simulink model "FSAC2021"  (R2014a)
settings: Solver=FixedStepDiscrete  StartTime=0.0  StopTime=inf  FixedStep=0.0005  RelTol=1e-3
model workspace (MAT data in the model file):
  MCOS : class17 (value not decoded)
  MCOS : class17 (value not decoded)
  MCOS : class17 (value not decoded)
  MCOS : class17 (value not decoded)
  MCOS : class17 (value not decoded)
  MCOS : class17 (value not decoded)
  MCOS : class17 (value not decoded)
  MCOS : class17 (value not decoded)
  MCOS : class17 (value not decoded)
  MCOS : class17 (value not decoded)
  MCOS : class17 (value not decoded)
  MCOS : class17 (value not decoded)
  MCOS : class17 (value not decoded)
  MCOS : class17 (value not decoded)
  MCOS : class17 (value not decoded)
  MCOS : class17 (value not decoded)
  MCOS : class17 (value not decoded)
  MCOS : class17 (value not decoded)
  MCOS : class17 (value not decoded)
  BUZZER_START = 1
  MCOS : class17 (value not decoded)
  MCOS : class17 (value not decoded)
  MCOS : class17 (value not decoded)
  MCOS : class17 (value not decoded)
  MCOS : class17 (value not decoded)
  MCOS : class17 (value not decoded)
  MCOS : class17 (value not decoded)
  MCOS : class17 (value not decoded)
  MCOS : class17 (value not decoded)
  MCOS : class17 (value not decoded)
  MCOS : class17 (value not decoded)
  MCOS : class17 (value not decoded)
  MCOS : class17 (value not decoded)
  MCOS : class17 (value not decoded)
  MCOS : class17 (value not decoded)
  MCOS : class17 (value not decoded)
  MCOS : class17 (value not decoded)
  MCOS : class17 (value not decoded)
  MCOS : class17 (value not decoded)
  MCOS : class17 (value not decoded)
  MCOS : class17 (value not decoded)
  MCOS : class17 (value not decoded)
  MCOS : class17 (value not decoded)
  MCOS : class17 (value not decoded)
  MCOS : class17 (value not decoded)
  MCOS : class17 (value not decoded)
  MCOS : class17 (value not decoded)
  MCOS : class17 (value not decoded)
  MCOS : class17 (value not decoded)
  MCOS : class17 (value not decoded)
  MCOS : class17 (value not decoded)
  MCOS : class17 (value not decoded)
  MCOS : class17 (value not decoded)
  MCOS : class17 (value not decoded)
  MCOS : class17 (value not decoded)
  MCOS : class17 (value not decoded)
  MCOS : class17 (value not decoded)
  MCOS : class17 (value not decoded)
  Brake = 11
  MCOS : class17 (value not decoded)
  MCOS : class17 (value not decoded)
  MCOS : class17 (value not decoded)
  MCOS : class17 (value not decoded)
  MCOS : class17 (value not decoded)
  MCOS : class17 (value not decoded)
  MCOS : class17 (value not decoded)
  MCOS : class17 (value not decoded)
  Sensor_Acc_b = 101.85
  Sensor_Acc_k = -0.0185
  Str_Sen_Orig_Angle = -341
  MCOS : class17 (value not decoded)
  Tire_D = 0.47
  T = 0.05
libraries: simulink x396, ec55xxlib x126
(part 2 of 17)

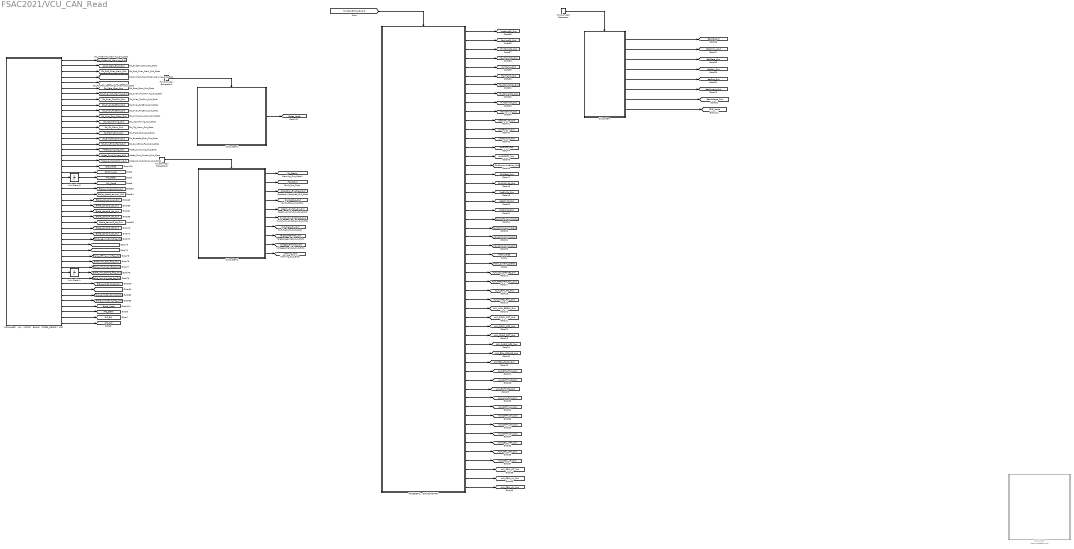
== system FSAC2021/VCU_CAN_Read ==
  DCAN_REC : Subsystem  Commented=on
  Function-Call Generator : simulink/Ports & Subsystems/Function-Call Generator  sample_time=0.1  numberOfIterations=1
  Function-Call Generator1 : simulink/Ports & Subsystems/Function-Call Generator  sample_time=0.5  numberOfIterations=1
  Function-Call Generator2 : simulink/Ports & Subsystems/Function-Call Generator  sample_time=0.1  numberOfIterations=1
  PCANA(RES、AMI、MOTEC、BRAKE、STEER_SENSOR、IPC) : Subsystem
  PCANB(BMS、DRIVE_MOTOR) : Subsystem
  Subsystem : Subsystem
  Subsystem1 : Subsystem
  Subsystem2 : Subsystem
  Unit Delay1 : UnitDelay  SampleTime=-1
  Unit Delay5 : UnitDelay  SampleTime=-1
  tag scope: ALM_AUX_FAIL_Out=global, ALM_BATT_DT_Out=global, ALM_BATT_DV_Out=global, ALM_BATT_OC_Out=global, ALM_BATT_OV_Out=global, ALM_BATT_UC_Out=global, ALM_BATT_UV_Out=global, ALM_BMU_FAIL_Out=global, ALM_BSU_FAULT_Out=global, ALM_BSU_OFFLINE_Out=global, ALM_CELL_IBK_Out=global, ALM_CELL_OT_Out=global, ALM_CELL_OV_Out=global, ALM_CELL_TBK_Out=global, ALM_CELL_UT_Out=global, ALM_CELL_UV_Out=global, ALM_CHRG_OCS_Out=global, ALM_CHRG_OCT_Out=global, ALM_DSCH_OCS_Out=global, ALM_DSCH_OCT_Out=global, ALM_HALL_BREAK_Out=global, ALM_HVREL_FAIL_Out=global, ALM_LEAK_OC_Out=global, ALM_PRECHRG_FAIL_Out=global, ALM_VCU_OFFLINE_Out=global, AMI_Node=global, AMI_State=global, BMS_Node=global, BatAlmLv_Out=global, BatCurrent_Out=global, BatLife_Out=global, BatSoc_Out=global, BatSoh_Out=global, BatState_Out=global, BatVoltage_Out=global, Brake_Node=global, Brake_cmd_fault_flag_Out=global, Brake_encoder_fault_sts_Out=global, Brake_go_origin_over_flag_Out=global, Brake_hd_fault_sts_Out=global, Brake_lowvolt_prtct_sts_Out=global, Brake_mtr_enable_flag_Out=global, Brake_mtr_goalpos_Out=global, Brake_mtr_origin_flag_Out=global, Brake_mtr_stop_flag_Out=global, Brake_offline_run_flag_Out=global, Brake_overcurrt_prtct_sts_Out=global, Brake_overheat_prtct_sts_Out=global, Brake_pos_enqual_Out=global, Brake_reg_rw_fault_flag_Out=global, Brake_sensor1_sts_Out=global, Brake_sensor2_sts_Out=global, Brake_sensor3_sts_Out=global, Brake_sensor4_sts_Out=global, Brake_sensor5_sts_Out=global, Brake_sensor6_sts_Out=global, Brake_speed_enqual_Out=global, ChrCommunication_Out=global, ChrReqCurr_Out=global, ChrReqVolt_Out=global, ChrState_Out=global, CoolingCtl_Out=global, Fault_Out=global, HeatingCtl_Out=global, IPC_Acc=global, IPC_Brk=global, IPC_Steer=global, MaxCellVoltNo_Out=global, MaxCellVolt_Out=global, MaxChrCurtLimit_Out=global, MaxChrPowerLimit_Out=global, MaxDisCurtLimit_Out=global, MaxDisPowerLimit_Out=global, MaxTempNo_Out=global, MaxTemp_Out=global, MinCellVoltNo_Out=global, MinCellVolt_Out=global, MinTempNo_Out=global, MinTemp_Out=global, Motec_Currt_Ang_Out=global, Motec_Currt_Current_Out=global, Motec_Currt_Position_Out=global, Motec_Node=global, Motor_Current_Speed=global, Motor_Node=global, NegRlyStr_Out=global, OnChrRlyStr_Out=global, Operation_Enabled_Out=global, PosRlyStr_Out=global, PreRlyStr_Out=global, Quick_Stop_Out=global, Ready_Switch_On_Out=global, StrSr_Node=global, Str_Curr_Error_Fault_Out=global, Str_Encoder_Error_Out=global, Str_Flash_Error_Out=global, Str_I2t_Alarm_Out=global, Str_I2t_Warning_Out=global, Str_Limit_Pos_Alarm_Out=global, Str_Over_PosError_Out=global, Str_Over_SpdError_Out=global, Str_Over_TopCurr_Out=global, Str_Overvolt_Warning_Out=global, Str_Para_Error_Out=global, Str_PwrMod_TempHigh_Alarm_Out=global, Str_PwrMod_TempHigh_Warning_Out=global, Str_Snr_Ang=global, Str_Spd_Over_Alam_Out=global, Str_Status=global, Str_System_Error_Out=global, Str_UnderVolt_Warning_Out=global, Switch_On_Disabled_Out=global, Swtiched_On_Out=global, Target_Reached_Out=global, Voltage_Enabled_Out=global, Warning_Out=global, chrOFFCC2_Out=global, chrONCC_Out=global, offChrRlyStr_Out=global
  wires:
  Subsystem/1(BATLIFE) -> [BatLife_Out]
  Subsystem/2(BATALM) -> [BatAlmLv_Out]
  Subsystem/3(BATSTATE) -> [BatState_Out]
  Subsystem/4(BATSOH) -> [BatSoh_Out]
  Subsystem/5(BATSOC) -> [BatSoc_Out]
  Subsystem/6(BATCURRENT) -> [BatCurrent_Out]
  Subsystem/7(BATVOLTAGLE) -> [BatVoltage_Out]
  Function-Call Generator/1 -> Subsystem/Trigger
  Subsystem/8(BMS_NODE) -> [BMS_Node]
  PCANB(BMS、DRIVE_MOTOR)/3(mintempno) -> [MinTempNo_Out]
  PCANB(BMS、DRIVE_MOTOR)/2(coolingctl) -> [CoolingCtl_Out]
  PCANB(BMS、DRIVE_MOTOR)/4(maxtempno) -> [MaxTempNo_Out]
  PCANB(BMS、DRIVE_MOTOR)/5(mintemp) -> [MinTemp_Out]
  PCANB(BMS、DRIVE_MOTOR)/1(heatingctl) -> [HeatingCtl_Out]
  PCANB(BMS、DRIVE_MOTOR)/6(maxtemp) -> [MaxTemp_Out]
  PCANB(BMS、DRIVE_MOTOR)/7(maxcellvoltno) -> [MaxCellVoltNo_Out]
  PCANB(BMS、DRIVE_MOTOR)/8(mincellvoltno) -> [MinCellVoltNo_Out]
  PCANB(BMS、DRIVE_MOTOR)/9(mincellvolt) -> [MinCellVolt_Out]
  PCANB(BMS、DRIVE_MOTOR)/10(maxcellvolt) -> [MaxCellVolt_Out]
  [FunCall_50ms_Duty8] -> PCANB(BMS、DRIVE_MOTOR)/Trigger
  PCANB(BMS、DRIVE_MOTOR)/11(offChrRlyStr_Out) -> [offChrRlyStr_Out]
  PCANB(BMS、DRIVE_MOTOR)/18(OnChrRlyStr_Out) -> [OnChrRlyStr_Out]
  PCANB(BMS、DRIVE_MOTOR)/14(chrONCC_Out) -> [chrONCC_Out]
  PCANB(BMS、DRIVE_MOTOR)/15(chrOFFCC2_Out) -> [chrOFFCC2_Out]
  PCANB(BMS、DRIVE_MOTOR)/16(ChrCommunication_Out) -> [ChrCommunication_Out]
  PCANB(BMS、DRIVE_MOTOR)/19(PreRlyStr_Out) -> [PreRlyStr_Out]
  PCANB(BMS、DRIVE_MOTOR)/13(ChrReqVolt_Out) -> [ChrReqVolt_Out]
  PCANB(BMS、DRIVE_MOTOR)/21(PosRlyStr_Out) -> [PosRlyStr_Out]
  PCANB(BMS、DRIVE_MOTOR)/20(NegRlyStr_Out) -> [NegRlyStr_Out]
  PCANB(BMS、DRIVE_MOTOR)/17(ChrState_Out) -> [ChrState_Out]
  PCANB(BMS、DRIVE_MOTOR)/12(ChrReqCurr_Out) -> [ChrReqCurr_Out]
  PCANB(BMS、DRIVE_MOTOR)/24(MaxDisCurtLimit_Out) -> [MaxDisCurtLimit_Out]
  PCANB(BMS、DRIVE_MOTOR)/23(MaxChrPowerLimit_Out) -> [MaxChrPowerLimit_Out]
  PCANB(BMS、DRIVE_MOTOR)/25(MaxChrCurtLimit_Out) -> [MaxChrCurtLimit_Out]
  PCANB(BMS、DRIVE_MOTOR)/22(MaxDisPowerLimit_Out) -> [MaxDisPowerLimit_Out]
  PCANB(BMS、DRIVE_MOTOR)/26(Motor_Node) -> [Motor_Node]
  PCANB(BMS、DRIVE_MOTOR)/27(Motor_Current_Speed) -> [Motor_Current_Speed]
  PCANB(BMS、DRIVE_MOTOR)/38(ALM_BSU_FAULT_Out) -> [ALM_BSU_FAULT_Out]
  PCANB(BMS、DRIVE_MOTOR)/37(ALM_BSU_OFFLINE_Out) -> [ALM_BSU_OFFLINE_Out]
  PCANB(BMS、DRIVE_MOTOR)/39(ALM_BMU_FAIL_Out) -> [ALM_BMU_FAIL_Out]
  PCANB(BMS、DRIVE_MOTOR)/40(ALM_BATT_UC_Out) -> [ALM_BATT_UC_Out]
  PCANB(BMS、DRIVE_MOTOR)/36(ALM_CHRG_OCS_Out) -> [ALM_CHRG_OCS_Out]
  PCANB(BMS、DRIVE_MOTOR)/35(ALM_CHRG_OCT_Out) -> [ALM_CHRG_OCT_Out]
  PCANB(BMS、DRIVE_MOTOR)/41(ALM_BATT_OC_Out) -> [ALM_BATT_OC_Out]
  PCANB(BMS、DRIVE_MOTOR)/34(ALM_DSCH_OCS_Out) -> [ALM_DSCH_OCS_Out]
  PCANB(BMS、DRIVE_MOTOR)/42(ALM_AUX_FAIL_Out) -> [ALM_AUX_FAIL_Out]
  PCANB(BMS、DRIVE_MOTOR)/43(ALM_BATT_UV_Out) -> [ALM_BATT_UV_Out]
  PCANB(BMS、DRIVE_MOTOR)/33(ALM_DSCH_OCT_Out) -> [ALM_DSCH_OCT_Out]
  PCANB(BMS、DRIVE_MOTOR)/32(ALM_HALL_BREAK_Out) -> [ALM_HALL_BREAK_Out]
  PCANB(BMS、DRIVE_MOTOR)/44(ALM_BATT_OV_Out) -> [ALM_BATT_OV_Out]
  PCANB(BMS、DRIVE_MOTOR)/31(ALM_HVREL_FAIL_Out) -> [ALM_HVREL_FAIL_Out]
  PCANB(BMS、DRIVE_MOTOR)/45(ALM_BATT_DT_Out) -> [ALM_BATT_DT_Out]
  PCANB(BMS、DRIVE_MOTOR)/46(ALM_BATT_DV_Out) -> [ALM_BATT_DV_Out]
  PCANB(BMS、DRIVE_MOTOR)/30(ALM_LEAK_OC_Out) -> [ALM_LEAK_OC_Out]
  PCANB(BMS、DRIVE_MOTOR)/47(ALM_CELL_TBK_Out) -> [ALM_CELL_TBK_Out]
  PCANB(BMS、DRIVE_MOTOR)/29(ALM_PRECHRG_FAIL_Out) -> [ALM_PRECHRG_FAIL_Out]
  PCANB(BMS、DRIVE_MOTOR)/48(ALM_CELL_IBK_Out) -> [ALM_CELL_IBK_Out]
  PCANB(BMS、DRIVE_MOTOR)/28(ALM_VCU_OFFLINE_Out) -> [ALM_VCU_OFFLINE_Out]
  PCANB(BMS、DRIVE_MOTOR)/49(ALM_CELL_UT_Out) -> [ALM_CELL_UT_Out]
  PCANB(BMS、DRIVE_MOTOR)/50(ALM_CELL_OT_Out) -> [ALM_CELL_OT_Out]
  PCANB(BMS、DRIVE_MOTOR)/51(ALM_CELL_UV_Out) -> [ALM_CELL_UV_Out]
  PCANB(BMS、DRIVE_MOTOR)/52(ALM_CELL_OV_Out) -> [ALM_CELL_OV_Out]
  Subsystem1/1(Motec_Node) -> [Motec_Node]
  Function-Call Generator1/1 -> Subsystem1/Trigger
  Subsystem2/2(Fault) -> [Fault_Out]
  Subsystem2/3(operation_enable) -> [Operation_Enabled_Out]
  Subsystem2/4(quick_stop) -> [Quick_Stop_Out]
  Subsystem2/5(ready_switch_on) -> [Ready_Switch_On_Out]
  Subsystem2/6(switch_on_disable) -> [Switch_On_Disabled_Out]
  Subsystem2/7(switch_on) -> [Swtiched_On_Out]
  Subsystem2/8(target_reached) -> [Target_Reached_Out]
  Subsystem2/9(voltagle_enable) -> [Voltage_Enabled_Out]
  Subsystem2/10(warning_out) -> [Warning_Out]
  Subsystem2/1(Str_Status) -> [Str_Status]
  Function-Call Generator2/1 -> Subsystem2/Trigger
  PCANA(RES、AMI、MOTEC、BRAKE、STEER_SENSOR、IPC)/16(Str_Curr_Error_Fault_Out) -> [Str_Curr_Error_Fault_Out]
  PCANA(RES、AMI、MOTEC、BRAKE、STEER_SENSOR、IPC)/15(Str_Encoder_Error_Out) -> [Str_Encoder_Error_Out]
  PCANA(RES、AMI、MOTEC、BRAKE、STEER_SENSOR、IPC)/14(Str_Flash_Error_Out) -> [Str_Flash_Error_Out]
  PCANA(RES、AMI、MOTEC、BRAKE、STEER_SENSOR、IPC)/13(Str_I2t_Alarm_Out) -> [Str_I2t_Alarm_Out]
  PCANA(RES、AMI、MOTEC、BRAKE、STEER_SENSOR、IPC)/12(Str_I2t_Warning_Out) -> [Str_I2t_Warning_Out]
  PCANA(RES、AMI、MOTEC、BRAKE、STEER_SENSOR、IPC)/11(Str_Limit_Pos_Alarm_Out) -> [Str_Limit_Pos_Alarm_Out]
  PCANA(RES、AMI、MOTEC、BRAKE、STEER_SENSOR、IPC)/10(Str_Over_PosError_Out) -> [Str_Over_PosError_Out]
  PCANA(RES、AMI、MOTEC、BRAKE、STEER_SENSOR、IPC)/9(Str_Over_SpdError_Out) -> [Str_Over_SpdError_Out]
  PCANA(RES、AMI、MOTEC、BRAKE、STEER_SENSOR、IPC)/8(Str_Over_TopCurr_Out) -> [Str_Over_TopCurr_Out]
  PCANA(RES、AMI、MOTEC、BRAKE、STEER_SENSOR、IPC)/7(Str_Overvolt_Warning_Out) -> [Str_Overvolt_Warning_Out]
  PCANA(RES、AMI、MOTEC、BRAKE、STEER_SENSOR、IPC)/6(Str_Para_Error_Out) -> [Str_Para_Error_Out]
  PCANA(RES、AMI、MOTEC、BRAKE、STEER_SENSOR、IPC)/5(Str_PwrMod_TempHigh_Alarm_Out) -> [Str_PwrMod_TempHigh_Alarm_Out]
  PCANA(RES、AMI、MOTEC、BRAKE、STEER_SENSOR、IPC)/4(Str_PwrMod_TempHigh_Warning_Out) -> [Str_PwrMod_TempHigh_Warning_Out]
  PCANA(RES、AMI、MOTEC、BRAKE、STEER_SENSOR、IPC)/3(Str_Spd_Over_Alam_Out) -> [Str_Spd_Over_Alam_Out]
  PCANA(RES、AMI、MOTEC、BRAKE、STEER_SENSOR、IPC)/2(Str_System_Error_Out) -> [Str_System_Error_Out]
  PCANA(RES、AMI、MOTEC、BRAKE、STEER_SENSOR、IPC)/1(Str_UnderVolt_Warning_Out) -> [Str_UnderVolt_Warning_Out]
  PCANA(RES、AMI、MOTEC、BRAKE、STEER_SENSOR、IPC)/17(Motec_Currt_Ang_Out) -> [Motec_Currt_Ang_Out]
  PCANA(RES、AMI、MOTEC、BRAKE、STEER_SENSOR、IPC)/18(Motec_Currt_Current_Out) -> [Motec_Currt_Current_Out]
  PCANA(RES、AMI、MOTEC、BRAKE、STEER_SENSOR、IPC)/19(Motec_Currt_Position_Out) -> [Motec_Currt_Position_Out]
  PCANA(RES、AMI、MOTEC、BRAKE、STEER_SENSOR、IPC)/20(StrSr_Node) -> [StrSr_Node]
  PCANA(RES、AMI、MOTEC、BRAKE、STEER_SENSOR、IPC)/21(StrSr_Snr_Ang) -> [Str_Snr_Ang]
  PCANA(RES、AMI、MOTEC、BRAKE、STEER_SENSOR、IPC)/22(AMI_State) -> Unit Delay5/1
  PCANA(RES、AMI、MOTEC、BRAKE、STEER_SENSOR、IPC)/23(AMI_Node) -> [AMI_Node]
  PCANA(RES、AMI、MOTEC、BRAKE、STEER_SENSOR、IPC)/44(Brake_cmd_fault_flag_Out) -> [Brake_cmd_fault_flag_Out]
  PCANA(RES、AMI、MOTEC、BRAKE、STEER_SENSOR、IPC)/43(Brake_encoder_fault_sts_Out) -> [Brake_encoder_fault_sts_Out]
  PCANA(RES、AMI、MOTEC、BRAKE、STEER_SENSOR、IPC)/42(Brake_go_origin_over_flag_Out) -> [Brake_go_origin_over_flag_Out]
  PCANA(RES、AMI、MOTEC、BRAKE、STEER_SENSOR、IPC)/41(Brake_hd_fault_sts_Out) -> [Brake_hd_fault_sts_Out]
  PCANA(RES、AMI、MOTEC、BRAKE、STEER_SENSOR、IPC)/40(Brake_lowvolt_prtct_sts_Out) -> [Brake_lowvolt_prtct_sts_Out]
  PCANA(RES、AMI、MOTEC、BRAKE、STEER_SENSOR、IPC)/39(Brake_mtr_enable_flag_Out) -> Unit Delay1/1
  PCANA(RES、AMI、MOTEC、BRAKE、STEER_SENSOR、IPC)/38(Brake_mtr_origin_flag_Out) -> [Brake_mtr_origin_flag_Out]
  PCANA(RES、AMI、MOTEC、BRAKE、STEER_SENSOR、IPC)/37(Brake_mtr_stop_flag_Out) -> [Brake_mtr_stop_flag_Out]
  PCANA(RES、AMI、MOTEC、BRAKE、STEER_SENSOR、IPC)/36(Brake_offline_run_flag_O) -> [Brake_offline_run_flag_Out]
  PCANA(RES、AMI、MOTEC、BRAKE、STEER_SENSOR、IPC)/35(Brake_overcurrt_prtct_sts_Out) -> [Brake_overcurrt_prtct_sts_Out]
  PCANA(RES、AMI、MOTEC、BRAKE、STEER_SENSOR、IPC)/34(Brake_overheat_prtct_sts_Out) -> [Brake_overheat_prtct_sts_Out]
  PCANA(RES、AMI、MOTEC、BRAKE、STEER_SENSOR、IPC)/33(Brake_reg_rw_fault_flag_Out) -> [Brake_reg_rw_fault_flag_Out]
  PCANA(RES、AMI、MOTEC、BRAKE、STEER_SENSOR、IPC)/32(Brake_sensor1_sts_Out) -> [Brake_sensor1_sts_Out]
  PCANA(RES、AMI、MOTEC、BRAKE、STEER_SENSOR、IPC)/31(Brake_sensor2_sts_Out) -> [Brake_sensor2_sts_Out]
  PCANA(RES、AMI、MOTEC、BRAKE、STEER_SENSOR、IPC)/30(Brake_sensor3_sts_Out) -> [Brake_sensor3_sts_Out]
  PCANA(RES、AMI、MOTEC、BRAKE、STEER_SENSOR、IPC)/29(Brake_sensor4_sts_Out) -> [Brake_sensor4_sts_Out]
  PCANA(RES、AMI、MOTEC、BRAKE、STEER_SENSOR、IPC)/28(Brake_sensor5_sts_Out) -> [Brake_sensor5_sts_Out]
  PCANA(RES、AMI、MOTEC、BRAKE、STEER_SENSOR、IPC)/27(Brake_sensor6_sts_Out) -> [Brake_sensor6_sts_Out]
  PCANA(RES、AMI、MOTEC、BRAKE、STEER_SENSOR、IPC)/26(Brake_pos_enqual_Out) -> [Brake_pos_enqual_Out]
  PCANA(RES、AMI、MOTEC、BRAKE、STEER_SENSOR、IPC)/25(Brake_speed_enqual_Out) -> [Brake_speed_enqual_Out]
  PCANA(RES、AMI、MOTEC、BRAKE、STEER_SENSOR、IPC)/24(Brake_mtr_goalpos_Out) -> [Brake_mtr_goalpos_Out]
  PCANA(RES、AMI、MOTEC、BRAKE、STEER_SENSOR、IPC)/45(Brk_Node) -> [Brake_Node]
  Unit Delay5/1 -> [AMI_State]
  Unit Delay1/1 -> [Brake_mtr_enable_flag_Out]
  PCANA(RES、AMI、MOTEC、BRAKE、STEER_SENSOR、IPC)/48(IPC_Acc) -> [IPC_Acc]
  PCANA(RES、AMI、MOTEC、BRAKE、STEER_SENSOR、IPC)/46(IPC_Steer) -> [IPC_Steer]
  PCANA(RES、AMI、MOTEC、BRAKE、STEER_SENSOR、IPC)/47(IPC_Brk) -> [IPC_Brk]

== system FSAC2021/VCU_KL_Read ==
  Read_VCU_AnaInput : Subsystem
  Read_VCU_DigInput : Subsystem
  Read_VCU_Freq(WheelSpeed) : Subsystem
  tag scope: ASMS=global, Acc_Lft_Disp_mv=global, Acc_Right_Disp_mv=global, Brk_Liquid_Prs_mv=global, Compare_Volt_mv=global, EBS_GAS_Prs_1_mv=global, EBS_GAS_Prs_2_mv=global, EBS_Rel_Switch=global, FL_WhlSpd_Hz=global, FR_WhlSpd_Hz=global, HVMS=global, HV_LIGHT=global, IMD_BENDER=global, LVMS=global, On_In_Switch=global, On_Out_Switch=global, RL_WhlSpd_Hz=global, RR_WhlSpd_Hz=global, START=global
  wires:
  [FunCall_50ms_Duty2] -> Read_VCU_Freq(WheelSpeed)/Trigger
  [FunCall_50ms_Duty6] -> Read_VCU_DigInput/Trigger
  [FunCall_50ms_Duty7] -> Read_VCU_AnaInput/Trigger
  Read_VCU_Freq(WheelSpeed)/1(RL_WhlSpd_Hz) -> [RL_WhlSpd_Hz], [FL_WhlSpd_Hz]
  Read_VCU_Freq(WheelSpeed)/2(RR_WhlSpd_Hz) -> [FR_WhlSpd_Hz], [RR_WhlSpd_Hz]
  Read_VCU_DigInput/1(LVMS) -> [LVMS]
  Read_VCU_DigInput/2(HVMS) -> [HVMS]
  Read_VCU_DigInput/3(ASMS) -> [ASMS]
  Read_VCU_DigInput/4(On_out_switch) -> [On_Out_Switch]
  Read_VCU_DigInput/5(Start) -> [START]
  Read_VCU_DigInput/6(On_in_switch) -> [On_In_Switch]
  Read_VCU_DigInput/7(HV_light) -> [HV_LIGHT]
  Read_VCU_DigInput/8(IMD_bender) -> [IMD_BENDER]
  Read_VCU_DigInput/9(EBS_Rel) -> [EBS_Rel_Switch]
  Read_VCU_AnaInput/6(EBS_GAS2) -> [EBS_GAS_Prs_2_mv]
  Read_VCU_AnaInput/5(EBS_GAS1) -> [EBS_GAS_Prs_1_mv]
  Read_VCU_AnaInput/4(BRK_LIQUID) -> [Brk_Liquid_Prs_mv]
  Read_VCU_AnaInput/3(COMPARE_VOLTAGLE) -> [Compare_Volt_mv]
  Read_VCU_AnaInput/2(ACC_RIGHT) -> [Acc_Right_Disp_mv]
  Read_VCU_AnaInput/1(ACC_LEFT) -> [Acc_Lft_Disp_mv]

== system FSAC2021/CAN_SEND/(BRK、STR、DRIVER) ==
  Brk_Mtr_GoalPos : Inport
  Acc_Cmd : Inport  Port=2
  BatVoltage_Out : Inport  Port=3
  Motor_Current_Speed : Inport  Port=4
  ASSI_State : Inport  Port=5
  vspd : Inport  Port=6
  BCU_MTR_MOVE_AB : Subsystem
  BCU_STATUS_READ : Subsystem
  CANTransmit3 : ec55xxlib/RapidECU_U2/07CANCommucation/CANTransmit  Commented=on  canmodule=A  canbuffer=58  canmessageid=358  canmessagetype=Standard(11-bit ID)  datalength=4  sampletime=0.05
  CANTransmit4 : ec55xxlib/RapidECU_U2/07CANCommucation/CANTransmit  canmodule=B  canbuffer=15  canmessageid=2197885092  canmessagetype=Extended(29-bit ID)  datalength=2  sampletime=0.05
  CANTransmit6 : ec55xxlib/RapidECU_U2/07CANCommucation/CANTransmit  canmodule=A  canbuffer=59  canmessageid=382  canmessagetype=Standard(11-bit ID)  datalength=2  sampletime=0.01
  CANTransmit7 : ec55xxlib/RapidECU_U2/07CANCommucation/CANTransmit  canmodule=A  canbuffer=60  canmessageid=1161  canmessagetype=Standard(11-bit ID)  datalength=8  sampletime=0.03
  Constant : Constant  Value=2
  Constant1 : Constant
  Data Type Conversion17 : DataTypeConversion
  MOTOR_SPEED_CONTROL : Subsystem
  MeaModule : ec55xxlib/RapidECU_U2/11Calibration/MeaModule  signal=To_MOTOR_OK
  MeaModule1 : ec55xxlib/RapidECU_U2/11Calibration/MeaModule  signal=ACC
  MeaModule2 : ec55xxlib/RapidECU_U2/11Calibration/MeaModule  signal=Read_BCU
  MeaModule3 : ec55xxlib/RapidECU_U2/11Calibration/MeaModule  signal=To_AMI_OK
  MeaModule4 : ec55xxlib/RapidECU_U2/11Calibration/MeaModule  signal=Vspd
  MeaModule5 : ec55xxlib/RapidECU_U2/11Calibration/MeaModule  signal=Motor_Spd
  MeaModule6 : ec55xxlib/RapidECU_U2/11Calibration/MeaModule  signal=Voltage
  MeaModule7 : ec55xxlib/RapidECU_U2/11Calibration/MeaModule  signal=ASSI_state
  Terminator3 : Terminator  Commented=on
  Terminator4 : Terminator
  Terminator6 : Terminator
  Terminator7 : Terminator
  To_AMI : Subsystem
  wires:
  Brk_Mtr_GoalPos/1 -> Data Type Conversion17/1
  CANTransmit3/1 -> Terminator3/1
  MOTOR_SPEED_CONTROL/1(output) -> CANTransmit4/1
  CANTransmit4/1 -> MeaModule/1
  Acc_Cmd/1 -> MeaModule1/1
  Data Type Conversion17/1 -> BCU_MTR_MOVE_AB/1(Brake_mtr_goalpos_in)
  MeaModule/1 -> Terminator4/1
  MeaModule1/1 -> MOTOR_SPEED_CONTROL/1(Drive_Speed_Control_in)
  Constant/1 -> BCU_STATUS_READ/1(status_reg_num_in)
  Constant1/1 -> BCU_STATUS_READ/2(status_reg_addr_start_in)
  BCU_STATUS_READ/1(output) -> CANTransmit6/1
  CANTransmit6/1 -> MeaModule2/1
  MeaModule2/1 -> Terminator6/1
  To_AMI/1(output) -> CANTransmit7/1
  CANTransmit7/1 -> MeaModule3/1
  BatVoltage_Out/1 -> MeaModule6/1
  Motor_Current_Speed/1 -> MeaModule5/1
  ASSI_State/1 -> MeaModule7/1
  vspd/1 -> MeaModule4/1
  MeaModule3/1 -> Terminator7/1
  MeaModule4/1 -> To_AMI/1(vspd_in)
  MeaModule5/1 -> To_AMI/2(mtr_rpm_in)
  MeaModule6/1 -> To_AMI/3(Battery_Volt_in)
  MeaModule7/1 -> To_AMI/4(assi_status_in)

== system FSAC2021/CAN_SEND/Subsystem ==
  CANTransmit5 : ec55xxlib/RapidECU_U2/07CANCommucation/CANTransmit  canmodule=B  canbuffer=56  canmessageid=2181107875  canmessagetype=Extended(29-bit ID)  datalength=8  sampletime=0.01
  MOTOR_READ_SPEED : Subsystem
  Terminator5 : Terminator
  wires:
  MOTOR_READ_SPEED/1(output) -> CANTransmit5/1
  CANTransmit5/1 -> Terminator5/1

== system FSAC2021/CAN_SEND/Subsystem1 ==
  Tmt_RPD01_CAN_FunCall : Inport
  Switch_On_Ctrl : Inport  Port=2
  Enable_Voltage_Ctrl : Inport  Port=3
  Quick_Stop_Ctrl : Inport  Port=4
  Enable_Operation_Ctrl : Inport  Port=5
  New_Set_Point_Ctrl : Inport  Port=6
  Abs_or_Rel_Ctrl : Inport  Port=7
  Halt_Ctrl : Inport  Port=8
  Position_set : Inport  Port=9
  Tmt_NMT_CAN_FunCall : Inport  Port=10
  NMT_nodeorder : Inport  Port=11
  NMT_nodectrl : Inport  Port=12
  Tmt_SDO_CAN_FunCall : Inport  Port=13
  Encoder_Msg_Data : Inport  Port=14
  Fault_Reset : Inport  Port=15
  assi_state : Inport  Port=16
  Brk_Mtr_Enbale : Subsystem  TreatAsAtomicUnit=on
  CANTransmit : ec55xxlib/RapidECU_U2/07CANCommucation/CANTransmit  canmodule=A  canbuffer=63  canmessageid=513  canmessagetype=Standard(11-bit ID)  datalength=6  sampletime=-1
  CANTransmit1 : ec55xxlib/RapidECU_U2/07CANCommucation/CANTransmit  canmodule=A  canbuffer=62  canmessageid=0  canmessagetype=Standard(11-bit ID)  datalength=2  sampletime=-1
  CANTransmit2 : ec55xxlib/RapidECU_U2/07CANCommucation/CANTransmit  canmodule=A  canbuffer=61  canmessageid=1537  canmessagetype=Standard(11-bit ID)  datalength=6  sampletime=-1
  Compare To Constant : simulink/Logic and Bit Operations/Compare To Constant  relop=>=  const=3  OutDataTypeStr=boolean
  Constant : Constant  Value=0  OutDataTypeStr=uint8
  Data Type Conversion{,1..16} (17 alike) : DataTypeConversion
  Demux : Demux  Outputs=6
  MOTEC_CONTROL : Subsystem
  MOTEC_ENCODER1 : Subsystem
  MOTEC_NMT : Subsystem
  MeaModule10 : ec55xxlib/RapidECU_U2/11Calibration/MeaModule  signal=ENCODER_SEND
  MeaModule8 : ec55xxlib/RapidECU_U2/11Calibration/MeaModule  signal=Metoc_Move
  MeaModule9 : ec55xxlib/RapidECU_U2/11Calibration/MeaModule  signal=MNT_SEND
  Switch : Switch  Criteria=u2 > Threshold
  Terminator : Terminator
  Terminator1 : Terminator
  Terminator2 : Terminator
  Unit Delay{,1..16} (17 alike) : UnitDelay  SampleTime=-1
  wires:
  CANTransmit/1 -> MeaModule8/1
  Halt_Ctrl/1 -> Unit Delay7/1
  Unit Delay3/1 -> Data Type Conversion5/1
  Unit Delay4/1 -> Data Type Conversion6/1
  Unit Delay5/1 -> Data Type Conversion7/1
  Unit Delay2/1 -> Data Type Conversion4/1
  Quick_Stop_Ctrl/1 -> Unit Delay2/1
  Abs_or_Rel_Ctrl/1 -> Unit Delay5/1
  New_Set_Point_Ctrl/1 -> Unit Delay4/1
  Enable_Voltage_Ctrl/1 -> Unit Delay1/1
  Enable_Operation_Ctrl/1 -> Unit Delay3/1
  Unit Delay1/1 -> Data Type Conversion3/1
  Unit Delay8/1 -> Data Type Conversion10/1
  Unit Delay7/1 -> Data Type Conversion9/1
  Switch_On_Ctrl/1 -> Unit Delay/1
  Unit Delay/1 -> Data Type Conversion2/1
  Data Type Conversion13/1 -> Unit Delay13/1
  Data Type Conversion12/1 -> Unit Delay12/1
  NMT_nodectrl/1 -> Unit Delay9/1
  Data Type Conversion/1 -> MOTEC_NMT/1(NMT_nodeorder_in)
  NMT_nodeorder/1 -> Unit Delay10/1
  Tmt_NMT_CAN_FunCall/1 -> MOTEC_NMT/Trigger
  Data Type Conversion1/1 -> MOTEC_NMT/2(NMT_nodectrl_in)
  CANTransmit1/1 -> MeaModule9/1
  Tmt_SDO_CAN_FunCall/1 -> MOTEC_ENCODER1/Trigger
  Encoder_Msg_Data/1 -> Demux/1
  Data Type Conversion16/1 -> Unit Delay16/1
  Unit Delay9/1 -> Data Type Conversion1/1
  Unit Delay10/1 -> Data Type Conversion/1
  Data Type Conversion14/1 -> Unit Delay14/1
  Demux/5 -> Data Type Conversion15/1
  CANTransmit2/1 -> MeaModule10/1
  Unit Delay6/1 -> Data Type Conversion8/1
  Data Type Conversion8/1 -> MOTEC_CONTROL/1(Fault_Reset_in)
  Data Type Conversion10/1 -> MOTEC_CONTROL/2(Position_set_in)
  Data Type Conversion3/1 -> MOTEC_CONTROL/8(Enable_Voltage_Ctrl_in)
  Data Type Conversion4/1 -> MOTEC_CONTROL/7(Quick_Stop_Ctrl_in)
  Data Type Conversion5/1 -> MOTEC_CONTROL/9(Enable_Operation_Ctrl_in)
  Position_set/1 -> Unit Delay8/1
  Data Type Conversion7/1 -> MOTEC_CONTROL/5(Abs_or_Rel_Ctrl_in)
  Data Type Conversion6/1 -> MOTEC_CONTROL/3(New_Pos_Set_in)
  Data Type Conversion2/1 -> MOTEC_CONTROL/6(Switch_On_Ctrl_in)
  Data Type Conversion9/1 -> MOTEC_CONTROL/4(Halt_Ctrl_in)
  Tmt_RPD01_CAN_FunCall/1 -> MOTEC_CONTROL/Trigger
  Demux/4 -> Data Type Conversion14/1
  MeaModule8/1 -> Terminator/1
  Data Type Conversion15/1 -> Unit Delay15/1
  Demux/6 -> Data Type Conversion16/1
  Demux/2 -> Data Type Conversion12/1
  MeaModule9/1 -> Terminator1/1
  Fault_Reset/1 -> Unit Delay6/1
  Data Type Conversion11/1 -> Unit Delay11/1
  Demux/1 -> Data Type Conversion11/1
  Demux/3 -> Data Type Conversion13/1
  MeaModule10/1 -> Terminator2/1
  MOTEC_CONTROL/1(output) -> CANTransmit/1
  MOTEC_NMT/1(output) -> CANTransmit1/1
  MOTEC_ENCODER1/1(output) -> CANTransmit2/1
  Unit Delay11/1 -> MOTEC_ENCODER1/1(Str_Encoder1_in)
  Unit Delay12/1 -> MOTEC_ENCODER1/2(Str_Encoder2_in)
  Unit Delay14/1 -> MOTEC_ENCODER1/4(Str_Encoder4_in)
  Unit Delay13/1 -> MOTEC_ENCODER1/3(Str_Encoder3_in)
  Unit Delay16/1 -> MOTEC_ENCODER1/6(Str_Encoder6_in)
  assi_state/1 -> Compare To Constant/1
  Compare To Constant/1 -> Switch/2
  Unit Delay15/1 -> Switch/3
  Switch/1 -> MOTEC_ENCODER1/5(Str_Encoder5_in)
  Constant/1 -> Switch/1

== system FSAC2021/Controller/200ms_Duty ==
  LED_Blue_Flag : Inport
  LED_Yellow_Flag : Inport  Port=2
  Buzzer_Flag : Inport  Port=3
  function : TriggerPort  TriggerType=function-call
  Light_Subsystem : Subsystem  TreatAsAtomicUnit=on
  Light_Subsystem1 : Subsystem  TreatAsAtomicUnit=on
  Light_Subsystem2 : Subsystem  TreatAsAtomicUnit=on
  Blue_Light_Pin : Outport
  Yellow_Light_Pin : Outport  Port=2
  Buzzer_Pin : Outport  Port=3
  Buzzer_Overflag : Outport  Port=4
  wires:
  LED_Yellow_Flag/1 -> Light_Subsystem1/1(Light_Status)
  Light_Subsystem1/1(Light_Output) -> Yellow_Light_Pin/1
  LED_Blue_Flag/1 -> Light_Subsystem/1(Light_Status)
  Light_Subsystem/1(Light_Output) -> Blue_Light_Pin/1
  Buzzer_Flag/1 -> Light_Subsystem2/1(Buzzer_Flag)
  Light_Subsystem2/1(Buzzer_Pin) -> Buzzer_Pin/1
  Light_Subsystem2/2(Buzzer_Overflag) -> Buzzer_Overflag/1

== system FSAC2021/Controller/50ms_Duty ==
  HV_LIGHT : Inport
  HVMS : Inport  Port=2
  ON_OUT : Inport  Port=3
  ON_IN : Inport  Port=4
  EBS_GAS_Prs_1_Val : Inport  Port=5
  EBS_GAS_Prs_2_Val : Inport  Port=6
  Brk_Liquid_Val : Inport  Port=7
  Veh_Spd : Inport  Port=8
  ASMS : Inport  Port=9
  LVMS : Inport  Port=10
  AMI_State : Inport  Port=11
  RES_EBS : Inport  Port=12
  RES_GO : Inport  Port=13
  START : Inport  Port=14
  Misson_Finished : Inport  Port=15
  Str_Sys_Error : Inport  Port=16
  Brk_Sys_Error : Inport  Port=17
  Sensor_Error : Inport  Port=18
  Acc_Sensor_Error : Inport  Port=19
  Res_Origin_Flag : Inport  Port=20
  Buzzer_Overflag : Inport  Port=21
  IPC_Str_Cmd : Inport  Port=22
  IPC_Brk_Cmd : Inport  Port=23
  IPC_Acc_Cmd : Inport  Port=24
  Res_Str_Cmd : Inport  Port=25
  Res_Brk_Cmd : Inport  Port=26
  Res_Acc_Cmd : Inport  Port=27
  EBS_Failure : Inport  Port=28
  IMD_Error : Inport  Port=29
  BMS_Error : Inport  Port=30
  Manual_Acc : Inport  Port=31
  Node_Lost : Inport  Port=32
  Compare_Volt_mv : Inport  Port=33
  Origin_Flag : Inport  Port=34
  Allow_Ctr_Flag : Inport  Port=35
  function : TriggerPort  TriggerType=function-call
  2 : Constant  Value=0  OutDataTypeStr=uint8
  3 : Constant  Value=0  OutDataTypeStr=uint8
  4 : Constant  Value=0  OutDataTypeStr=uint8
  48Battry_Judge : Subsystem
  AS_Machine : Stateflow chart  TreatAsAtomicUnit=on
  Constant : Constant  OutDataTypeStr=uint8  LockScale=on
  Constant1 : Constant  OutDataTypeStr=uint8
  Constant2 : Constant  OutDataTypeStr=uint8  LockScale=on
  Constant3 : Constant  Value=0
  EBS_Judge : Subsystem
  "HV_Judge " : Subsystem
  Lights_Select : Subsystem
  MeaModule : ec55xxlib/RapidECU_U2/11Calibration/MeaModule  signal=TS_Flag
  MeaModule1 : ec55xxlib/RapidECU_U2/11Calibration/MeaModule  signal=EBS_Status
  MeaModule3 : ec55xxlib/RapidECU_U2/11Calibration/MeaModule  signal=RES_EBS
  MeaModule5 : ec55xxlib/RapidECU_U2/11Calibration/MeaModule  signal=AMI_State
  R2D_Judge : Subsystem
  Safety_Relay_Judge : Subsystem
  Subsystem : Subsystem
  Unit Delay5 : UnitDelay  SampleTime=-1
  Visuality Check : Subsystem  TreatAsAtomicUnit=on
  Blue_Light : Outport
  Yellow_Light : Outport  Port=2
  Buzzer : Outport  Port=3
  Safety_Relay_Pin : Outport  Port=4
  Relay_48V_Pin : Outport  Port=5
  VCU_Valve : Outport  Port=6
  R2D_Pin : Outport  Port=7
  Str_Ctr : Outport  Port=8
  Brk_Ctr : Outport  Port=9
  Acc_Ctr : Outport  Port=10
  ASSI_State : Outport  Port=11
  Trig_EBS_Flg_Out : Outport  Port=12
  IMD_Light_Sts : Outport  Port=13
  EBS_Light_Sts : Outport  Port=14
  BMS_Light_Sts : Outport  Port=15
  TS_Flag : Outport  Port=16
  wires:
  HV_LIGHT/1 -> "HV_Judge "/1(HV_LIGHT)
  HVMS/1 -> "HV_Judge "/2(HVMS)
  EBS_GAS_Prs_2_Val/1 -> EBS_Judge/2(EBS_GAS_Prs_2_Val)
  EBS_GAS_Prs_1_Val/1 -> EBS_Judge/1(EBS_GAS_Prs_1_Val)
  EBS_Judge/1(EBS_Status) -> MeaModule1/1, Trig_EBS_Flg_Out/1
  ASMS/1 -> AS_Machine/4(ASMS)
  LVMS/1 -> AS_Machine/5(LVMS)
  AMI_State/1 -> MeaModule5/1
  ON_OUT/1 -> "HV_Judge "/3(ON_OUT)
  AS_Machine/4(Safety_Circuit_Relay) -> Safety_Relay_Judge/1(Finish_State_Safety_Relay)
  AS_Machine/2(Yellow_Light) -> Yellow_Light/1
  AS_Machine/5(System_48V_Relay) -> 48Battry_Judge/3(AS_48V_Relay)
  AS_Machine/1(Blue_Light) -> Blue_Light/1
  AS_Machine/3(Buzzer) -> Buzzer/1
  AS_Machine/7(VCU_Valve) -> VCU_Valve/1
  AS_Machine/8(R2D) -> R2D_Judge/1(AS_R2D)
  Buzzer_Overflag/1 -> AS_Machine/11(Buzzer_Overflag)
  ON_IN/1 -> "HV_Judge "/4(ON_IN)
  RES_EBS/1 -> MeaModule3/1
  Safety_Relay_Judge/1(Safety_Cir_Relay_Pin) -> Safety_Relay_Pin/1
  R2D_Judge/1(R2D_Pin) -> R2D_Pin/1
  Acc_Sensor_Error/1 -> R2D_Judge/2(Acc_Sensor_Error)
  48Battry_Judge/1(Relay_48V_Pin) -> Relay_48V_Pin/1
  [AMI_Duty] -> Subsystem/2(AMI_Duty)
  IPC_Str_Cmd/1 -> Subsystem/6(IPC_Str_Cmd)
  IPC_Brk_Cmd/1 -> Subsystem/5(IPC_Brk_Cmd)
  IPC_Acc_Cmd/1 -> Subsystem/3(IPC_Acc_Cmd)
  Subsystem/1(Str_Ctr) -> Str_Ctr/1
  Subsystem/2(Brk_Ctr) -> Brk_Ctr/1
  EBS_Failure/1 -> [EBS_Failure]
  Brk_Liquid_Val/1 -> EBS_Judge/3(Brk_Liquid_Prs_Val)
  Visuality Check/1(Visual_Lights_Vector) -> Lights_Select/1(Visual_Lights_Vetor)
  Visuality Check/2(Visual_Flag) -> Lights_Select/2(Visual_Flag)
  IMD_Error/1 -> Lights_Select/3(IMD_Error)
  [EBS_Failure] -> Lights_Select/4(EBS_Error)
  BMS_Error/1 -> Lights_Select/5(BMS_Error)
  Lights_Select/2(EBS_Light_Sts) -> EBS_Light_Sts/1
  Lights_Select/1(IMD_Light_Sts) -> IMD_Light_Sts/1
  Lights_Select/3(BMS_Light_Sts) -> BMS_Light_Sts/1
  AS_Machine/10(Visuality_Check()) -> Visuality Check/Trigger
  Manual_Acc/1 -> Subsystem/1(Manual_Acc_Cmd)
  [EBS_Failure] -> Subsystem/4(EBS_Failure)
  AS_Machine/6(ASSI_State) -> ASSI_State/1
  MeaModule3/1 -> [RES_EBS]
  2/1 -> Safety_Relay_Judge/2(RES_EBS)
  Str_Sys_Error/1 -> Safety_Relay_Judge/3(Str_Sys_Error)
  Brk_Sys_Error/1 -> Safety_Relay_Judge/4(Brk_Sys_Error)
  3/1 -> Safety_Relay_Judge/5(Sensor_Error)
  Constant/1 -> AS_Machine/2(EBS_Flag)
  Veh_Spd/1 -> AS_Machine/3(Veh_Spd)
  MeaModule5/1 -> [AMI_Duty], AS_Machine/6(AMI_State)
  MeaModule/1 -> AS_Machine/1(TS_Flag)
  Compare_Volt_mv/1 -> "HV_Judge "/5(Compare_Volt_mv)
  "HV_Judge "/1(TS_Flag) -> MeaModule/1, TS_Flag/1
  Constant1/1 -> AS_Machine/12(Res_Origin_Flag)
  START/1 -> AS_Machine/8(Res_GO), AS_Machine/9(START_Flag)
  Origin_Flag/1 -> Subsystem/7(origin_flag)
  Subsystem/3(Mission_Flag) -> Unit Delay5/1
  [Mission_Flag] -> AS_Machine/10(Misson_Finished)
  Unit Delay5/1 -> [Mission_Flag]
  Constant2/1 -> AS_Machine/7(Res_EBS)
  Allow_Ctr_Flag/1 -> Subsystem/8(Allow_Ctr_Flag)
  Subsystem/4(Acc_Ctr) -> Acc_Ctr/1
  4/1 -> Safety_Relay_Judge/6(Node_Lost)
  Constant3/1 -> Safety_Relay_Judge/7(EBS_Failure)

== system FSAC2021/Controller/BCU_Controller ==
  note: 任何控制源禁止在Allow_Ctrl_Flg未置1的时候控制车辆
  Brk_Cmd : Inport
  Brk_Mtr_Enable_Flg : Inport  Port=2
  ASSI_State : Inport  Port=3
  function : TriggerPort  TriggerType=function-call
  BCU_Strategy : Stateflow chart
  Brk_Move : Subsystem
  Constant1 : Constant
  MeaModule : ec55xxlib/RapidECU_U2/11Calibration/MeaModule  signal=Brk_Enable_Flag
  Allow_Ctrl_Flg : Outport
  Brk_Mtr_Origin_funCall : Outport  Port=2
  Brk_Mtr_Enable_funCall : Outport  Port=3
  Brk_Mtr_GoalPos : Outport  Port=4
  wires:
  Brk_Mtr_Enable_Flg/1 -> MeaModule/1
  Constant1/1 -> BCU_Strategy/3(Brk_Mtr_Origin_Flag)
  BCU_Strategy/2(Brk_Ctrl_State) -> Brk_Move/1(Brk_Ctrl_State)
  ASSI_State/1 -> BCU_Strategy/2(ASSI_State)
  BCU_Strategy/1(Allow_Ctrl_Flg) -> Allow_Ctrl_Flg/1
  BCU_Strategy/3(Brk_Mtr_BackOrigin()) -> Brk_Mtr_Origin_funCall/1
  BCU_Strategy/4(Brk_Mtr_Enable()) -> Brk_Mtr_Enable_funCall/1
  Brk_Move/1(Brk_Mtr_GoalPos) -> Brk_Mtr_GoalPos/1
  Brk_Cmd/1 -> Brk_Move/2(Brk_Cmd)
  MeaModule/1 -> BCU_Strategy/1(Brk_Mtr_Enable_Flg)

== system FSAC2021/Controller/SteerCtr ==
  Str_Snr_Ang : Inport
  Steer_Cmd : Inport  Port=2
  Str_Status : Inport  Port=3
  ASSI_State : Inport  Port=4
  function : TriggerPort  TriggerType=function-call
  Chart : Stateflow chart  SystemSampleTime=0.01
  Data Type Conversion{,1..3} (4 alike) : DataTypeConversion
  MeaModule : ec55xxlib/RapidECU_U2/11Calibration/MeaModule  signal=Back_Angle
  MeaModule1 : ec55xxlib/RapidECU_U2/11Calibration/MeaModule  signal=enflag
  MeaModule2 : ec55xxlib/RapidECU_U2/11Calibration/MeaModule  signal=flag
  MeaModule3 : ec55xxlib/RapidECU_U2/11Calibration/MeaModule  signal=Str
  Subsystem3 : Subsystem
  Terminator : Terminator
  Terminator1 : Terminator
  NMT_nodeorder : Outport
  NMT_nodectrl : Outport  Port=2
  Enable_Operation_Ctrl : Outport  Port=3
  Quick_Stop_Ctrl : Outport  Port=4
  Enable_Voltage_Ctrl : Outport  Port=5
  Halt_Ctrl : Outport  Port=6
  Switch_On_Ctrl : Outport  Port=7
  Abs_or_Rel_Ctrl : Outport  Port=8
  New_Set_Point_Ctrl : Outport  Port=9
  Position_set : Outport  Port=10
  Encoder_Msg_Data : Outport  Port=11
  TmtNNMTCAN : Outport  Port=12
  TmtRPDO1CAN : Outport  Port=13
  TmtSDOCAN : Outport  Port=14
  Original_Flag : Outport  Port=15
  Fault_Reset : Outport  Port=16
  wires:
  Str_Status/1 -> Data Type Conversion1/1
  Data Type Conversion3/1 -> Subsystem3/1(In1)
  ASSI_State/1 -> Data Type Conversion/1
  Data Type Conversion2/1 -> MeaModule3/1
  Data Type Conversion/1 -> Chart/3(ASSI_State)
  Data Type Conversion1/1 -> Chart/4(Str_Status)
  Chart/1(NMT_nodeorder) -> NMT_nodeorder/1
  Chart/2(NMT_nodectrl) -> NMT_nodectrl/1
  Chart/3(Enable_Operation_Ctrl) -> Enable_Operation_Ctrl/1
  Chart/4(Quick_Stop_Ctrl) -> Quick_Stop_Ctrl/1
  Chart/5(Enable_Voltage_Ctrl) -> Enable_Voltage_Ctrl/1
  Chart/6(Halt_Ctrl) -> Halt_Ctrl/1
  Chart/7(Switch_On_Ctrl) -> Switch_On_Ctrl/1
  Chart/8(Abs_or_Rel_Ctrl) -> Abs_or_Rel_Ctrl/1
  Chart/9(New_Set_Point_Ctrl) -> New_Set_Point_Ctrl/1
  Chart/11(Encoder_Msg_Data) -> Encoder_Msg_Data/1
  Chart/12(Original_Flag) -> Original_Flag/1
  Chart/16(TmtNMTCAN()) -> TmtNNMTCAN/1
  Chart/17(TmtRPDO1CAN()) -> TmtRPDO1CAN/1
  Chart/18(TmtSDOCAN()) -> TmtSDOCAN/1
  Subsystem3/1(Out1) -> MeaModule/1
  MeaModule/1 -> Chart/1(Origin_Back_Angle)
  Str_Snr_Ang/1 -> Data Type Conversion3/1
  Chart/13(Fault_Resrt) -> Fault_Reset/1
  Chart/10(Position_set) -> Position_set/1
  Chart/14(flag) -> MeaModule2/1
  MeaModule2/1 -> Terminator/1
  MeaModule3/1 -> Chart/2(Steer_Go_Angle)
  Chart/15(enflag) -> MeaModule1/1
  MeaModule1/1 -> Terminator1/1
  Steer_Cmd/1 -> Data Type Conversion2/1

== system FSAC2021/DIAG/DIAG ==
  Acc_Lft_Disp_mv : Inport
  Acc_Right_Disp_mv : Inport  Port=2
  Brk_Liquid_Prs_mv : Inport  Port=3
  EBS_GAS_Prs_1_mv : Inport  Port=4
  EBS_GAS_Prs_2_mv : Inport  Port=5
  Str_UnderVolt_Warning_Out : Inport  Port=6
  Str_System_Error_Out : Inport  Port=7
  Str_Limit_Pos_Alarm_Out : Inport  Port=8
  Str_I2t_Warning_Out : Inport  Port=9
  Str_I2t_Alarm_Out : Inport  Port=10
  Str_Flash_Error_Out : Inport  Port=11
  Str_Encoder_Error_Out : Inport  Port=12
  Str_Curr_Error_Fault_Out : Inport  Port=13
  Str_Spd_Over_Alam_Out : Inport  Port=14
  Str_PwrMod_TempHigh_Warning_Out : Inport  Port=15
  Str_PwrMod_TempHigh_Alarm_Out : Inport  Port=16
  Str_Para_Error_Out : Inport  Port=17
  Str_Overvolt_Warning_Out : Inport  Port=18
  Str_Over_TopCurr_Out : Inport  Port=19
  Str_Over_SpdError_Out : Inport  Port=20
  Str_Over_PosError_Out : Inport  Port=21
  Brake_reg_rw_fault_flag_Out : Inport  Port=22
  Brake_overheat_prtct_sts_Out : Inport  Port=23
  Brake_overcurrt_prtct_sts_Out : Inport  Port=24
  Brake_lowvolt_prtct_sts_Out : Inport  Port=25
  Brake_hd_fault_sts_Out : Inport  Port=26
  Brake_encoder_fault_sts_Out : Inport  Port=27
  Brake_cmd_fault_flag_Out : Inport  Port=28
  Remote_Steer_Error_Out : Inport  Port=29
  Remote_GO_Error_Out : Inport  Port=30
  Remote_EBS_Error_Out : Inport  Port=31
  Remote_Brake_Error_Out : Inport  Port=32
  Remote_Acc_Error_Out : Inport  Port=33
  Brake_Node : Inport  Port=34
  AMI_Node : Inport  Port=35
  StrSr_Node : Inport  Port=36
  Relay_48V : Inport  Port=37
  RES_Node : Inport  Port=38
  BMS_Node : Inport  Port=39
  ALM_BATT_OC_Out1 : Inport  Port=40
  Motor_Node : Inport  Port=41
  ALM_AUX_FAIL_Out1 : Inport  Port=42
  ALM_BATT_UV_Out1 : Inport  Port=43
  ALM_BATT_OV_Out1 : Inport  Port=44
  ALM_BATT_DT_Out1 : Inport  Port=45
  ALM_BATT_DV_Out1 : Inport  Port=46
  ALM_CELL_TBK_Out1 : Inport  Port=47
  ALM_CELL_IBK_Out1 : Inport  Port=48
  ALM_CELL_UT_Out1 : Inport  Port=49
  ALM_CELL_OT_Out1 : Inport  Port=50
  ALM_CELL_UV_Out1 : Inport  Port=51
  ALM_CELL_OV_Out1 : Inport  Port=52
  ALM_BATT_UC_Out1 : Inport  Port=53
  ALM_PRECHRG_FAIL_Out1 : Inport  Port=54
  ALM_LEAK_OC_Out1 : Inport  Port=55
  ALM_HVREL_FAIL_Out1 : Inport  Port=56
  ALM_HALL_BREAK_Out1 : Inport  Port=57
  ALM_BSU_OFFLINE_Out1 : Inport  Port=58
  ALM_BSU_FAULT_Out1 : Inport  Port=59
  ALM_BMU_FAIL_Out1 : Inport  Port=60
  "IMD_BMS " : Inport  Port=61
  "IMD_BENDER " : Inport  Port=62
  Motec_Node : Inport  Port=63
  Compare_Volt_mv : Inport  Port=64
  ASSI_State : Inport  Port=65
  function : TriggerPort  TriggerType=function-call
  Analog_Sensor_Diag : Subsystem
  BMS_Diag : Subsystem
  Brake_System_Diag : Subsystem
  CAN_NODE_LOSTCOM : Subsystem
  EBS_Diag : Subsystem
  Res_Diag : Subsystem
  Steer_System_Diag : Subsystem
  TS_Diag : Subsystem
  TS_Diag1 : Subsystem
  Acc_Lft_Error : Outport
  Acc_Right_Disp_Error : Outport  Port=2
  Brk_Liquid_Prs_Error : Outport  Port=3
  Sensor_Error : Outport  Port=4
  EBS_GAP_pRS_1_Error : Outport  Port=5
  EBS_GAP_pRS_2_Error : Outport  Port=6
  Str_Sys_Error : Outport  Port=7
  Brk_Sys_Error : Outport  Port=8
  RES_Error : Outport  Port=9
  Node_Lost_Flag : Outport  Port=10
  TS_Error : Outport  Port=11
  EBS_Failure : Outport  Port=12
  "BMS_Error " : Outport  Port=13
  IMD_Error : Outport  Port=14
  wires:
  Str_UnderVolt_Warning_Out/1 -> Steer_System_Diag/1(Str_UnderVolt_Warning_Out)
  Str_System_Error_Out/1 -> Steer_System_Diag/2(Str_System_Error_Out)
  Str_Spd_Over_Alam_Out/1 -> Steer_System_Diag/3(Str_Limit_Pos_Alarm_Out)
  Str_PwrMod_TempHigh_Warning_Out/1 -> Steer_System_Diag/4(Str_I2t_Warning_Out)
  Str_PwrMod_TempHigh_Alarm_Out/1 -> Steer_System_Diag/5(Str_I2t_Alarm_Out)
  Str_Overvolt_Warning_Out/1 -> Steer_System_Diag/7(Str_Encoder_Error_Out)
  Str_Over_TopCurr_Out/1 -> Steer_System_Diag/8(Str_Curr_Error_Fault_Out)
  Str_Para_Error_Out/1 -> Steer_System_Diag/6(Str_Flash_Error_Out)
  Str_Over_SpdError_Out/1 -> Steer_System_Diag/9(Str_Spd_Over_Alam_Out)
  Str_Over_PosError_Out/1 -> Steer_System_Diag/10(Str_PwrMod_TempHigh_Warning_Out)
  Str_Limit_Pos_Alarm_Out/1 -> Steer_System_Diag/11(Str_PwrMod_TempHigh_Alarm_Out)
  Str_I2t_Warning_Out/1 -> Steer_System_Diag/12(Str_Para_Error_Out)
  Str_I2t_Alarm_Out/1 -> Steer_System_Diag/13(Str_Overvolt_Warning_Out)
  Str_Flash_Error_Out/1 -> Steer_System_Diag/14(Str_Over_TopCurr_Out)
  Str_Encoder_Error_Out/1 -> Steer_System_Diag/15(Str_Over_SpdError_Out)
  Str_Curr_Error_Fault_Out/1 -> Steer_System_Diag/16(Str_Over_PosError_Out)
  Steer_System_Diag/1(Str_Sys_Error) -> Str_Sys_Error/1
  Brake_overcurrt_prtct_sts_Out/1 -> Brake_System_Diag/3(Brake_overcurrt_prtct_sts_Out)
  Brake_overheat_prtct_sts_Out/1 -> Brake_System_Diag/2(Brake_overheat_prtct_sts_Out)
  Brake_lowvolt_prtct_sts_Out/1 -> Brake_System_Diag/4(Brake_lowvolt_prtct_sts_Out)
  Brake_reg_rw_fault_flag_Out/1 -> Brake_System_Diag/1(Brake_reg_rw_fault_flag_Out)
  Brake_hd_fault_sts_Out/1 -> Brake_System_Diag/5(Brake_hd_fault_sts_Out)
  Brake_encoder_fault_sts_Out/1 -> Brake_System_Diag/6(Brake_encoder_fault_sts_Out)
  Brake_cmd_fault_flag_Out/1 -> Brake_System_Diag/7(Brake_cmd_fault_flag_Out)
  Brake_System_Diag/1(Brk_Sys_Error) -> Brk_Sys_Error/1
  Acc_Right_Disp_mv/1 -> Analog_Sensor_Diag/2(Acc_Right_Disp_mv)
  Brk_Liquid_Prs_mv/1 -> Analog_Sensor_Diag/3(Brk_Liquid_Prs_mv)
  Acc_Lft_Disp_mv/1 -> Analog_Sensor_Diag/1(Acc_Lft_Disp_mv)
  Analog_Sensor_Diag/3(Brk_Liquid_Prs_Error) -> Brk_Liquid_Prs_Error/1
  Analog_Sensor_Diag/1(Acc_Lft_Error) -> Acc_Lft_Error/1
  Analog_Sensor_Diag/2(Acc_Right_Disp_Error) -> Acc_Right_Disp_Error/1
  Analog_Sensor_Diag/4(Sensor_Error) -> Sensor_Error/1
  Res_Diag/1(RES_Error) -> RES_Error/1
  Remote_Steer_Error_Out/1 -> Res_Diag/1(Remote_Steer_Error_Out)
  Remote_GO_Error_Out/1 -> Res_Diag/2(Remote_GO_Error_Out)
  Remote_EBS_Error_Out/1 -> Res_Diag/3(Remote_EBS_Error_Out)
  Remote_Brake_Error_Out/1 -> Res_Diag/4(Remote_Brake_Error_Out)
  Remote_Acc_Error_Out/1 -> Res_Diag/5(Remote_Acc_Error_Out)
  CAN_NODE_LOSTCOM/1(Node_Lost_Flag) -> Node_Lost_Flag/1
  TS_Diag/1(TS_Error) -> TS_Error/1
  Analog_Sensor_Diag/5(EBS_GAP_pRS_1_Error) -> EBS_GAP_pRS_1_Error/1
  EBS_GAS_Prs_1_mv/1 -> EBS_Diag/2(EBS_GAS_Prs_1_Val), Analog_Sensor_Diag/4(EBS_GAS_Prs_1_mv)
  EBS_GAS_Prs_2_mv/1 -> EBS_Diag/3(EBS_GAS_Prs_2_Val), Analog_Sensor_Diag/5(EBS_GAS_Prs_2_mv)
  EBS_Diag/1(EBS_Failuer_Flag) -> EBS_Failure/1
  ASSI_State/1 -> EBS_Diag/1(ASSI_State), TS_Diag/1(ASSI_State), CAN_NODE_LOSTCOM/9(ASSI_State)
  Analog_Sensor_Diag/6(EBS_GAP_pRS_2_Error) -> EBS_GAP_pRS_2_Error/1
  ALM_BATT_OC_Out1/1 -> BMS_Diag/1(ALM_BATT_OC_Out1)
  ALM_AUX_FAIL_Out1/1 -> BMS_Diag/2(ALM_AUX_FAIL_Out1)
  ALM_BATT_UV_Out1/1 -> BMS_Diag/3(ALM_BATT_UV_Out1)
  ALM_BATT_OV_Out1/1 -> BMS_Diag/4(ALM_BATT_OV_Out1)
  ALM_BATT_DT_Out1/1 -> BMS_Diag/5(ALM_BATT_DT_Out1)
  ALM_BATT_DV_Out1/1 -> BMS_Diag/6(ALM_BATT_DV_Out1)
  ALM_CELL_TBK_Out1/1 -> BMS_Diag/7(ALM_CELL_TBK_Out1)
  ALM_CELL_IBK_Out1/1 -> BMS_Diag/8(ALM_CELL_IBK_Out1)
  ALM_CELL_UT_Out1/1 -> BMS_Diag/9(ALM_CELL_UT_Out1)
  ALM_CELL_OT_Out1/1 -> BMS_Diag/10(ALM_CELL_OT_Out1)
  ALM_CELL_UV_Out1/1 -> BMS_Diag/11(ALM_CELL_UV_Out1)
  ALM_CELL_OV_Out1/1 -> BMS_Diag/12(ALM_CELL_OV_Out1)
  ALM_BATT_UC_Out1/1 -> BMS_Diag/13(ALM_BATT_UC_Out1)
  ALM_PRECHRG_FAIL_Out1/1 -> BMS_Diag/14(ALM_PRECHRG_FAIL_Out1)
  ALM_LEAK_OC_Out1/1 -> BMS_Diag/15(ALM_LEAK_OC_Out1)
  ALM_HVREL_FAIL_Out1/1 -> BMS_Diag/16(ALM_HVREL_FAIL_Out1)
  ALM_HALL_BREAK_Out1/1 -> BMS_Diag/17(ALM_HALL_BREAK_Out1)
  ALM_BSU_OFFLINE_Out1/1 -> BMS_Diag/18(ALM_BSU_OFFLINE_Out1)
  ALM_BSU_FAULT_Out1/1 -> BMS_Diag/19(ALM_BSU_FAULT_Out1)
  ALM_BMU_FAIL_Out1/1 -> BMS_Diag/20(ALM_BMU_FAIL_Out1)
  BMS_Diag/1("BMS_Error ") -> "BMS_Error "/1
  "IMD_BENDER "/1 -> TS_Diag1/2("IMD_BENDER ")
  "IMD_BMS "/1 -> TS_Diag1/1("IMD_BMS ")
  TS_Diag1/1(IMD_Error) -> IMD_Error/1
  Brake_Node/1 -> CAN_NODE_LOSTCOM/1(Brake_Node)
  Motor_Node/1 -> CAN_NODE_LOSTCOM/6(Motor_Node)
  StrSr_Node/1 -> CAN_NODE_LOSTCOM/2(StrSr_Node)
  RES_Node/1 -> CAN_NODE_LOSTCOM/4(RES_Node)
  BMS_Node/1 -> CAN_NODE_LOSTCOM/5(BMS_Node)
  Relay_48V/1 -> CAN_NODE_LOSTCOM/3(48V_Relay)
  Motec_Node/1 -> CAN_NODE_LOSTCOM/7(Motec_Node)
  Compare_Volt_mv/1 -> TS_Diag/2(Compare_Volt_mv)
  AMI_Node/1 -> CAN_NODE_LOSTCOM/8(AMI_Node)

== system FSAC2021/I//O_OutPut/Subsystem ==
  Blue_Light_Pin : Inport
  Yellow_Light_Pin : Inport  Port=2
  Buzzer_pin : Inport  Port=3
  Safety_Relay_Pin : Inport  Port=4
  Relay_48V_Pin : Inport  Port=5
  R2D_pin : Inport  Port=6
  VCU_valve : Inport  Port=7
  IMD_Light : Inport  Port=8
  EBS_Light : Inport  Port=9
  BMS_Light : Inport  Port=10
  function : TriggerPort  TriggerType=function-call
  48V_Relay : ec55xxlib/RapidECU_U2/04PowerDriverSwitch/PowerDriverSwitch  channel=59: O_PWM2_LS1A8  sampletime=-1
  Blue_Pin : ec55xxlib/RapidECU_U2/04PowerDriverSwitch/PowerDriverSwitch  channel=114: O_PWM9_HS2A9  sampletime=-1
  Buzzer_Pin : ec55xxlib/RapidECU_U2/04PowerDriverSwitch/PowerDriverSwitch  channel=117: O_PWM11_HS2A9  sampletime=-1
  Data Type Conversion{,1..6,8..10} (10 alike) : DataTypeConversion  OutDataTypeStr=boolean
  MeaModule : ec55xxlib/RapidECU_U2/11Calibration/MeaModule  signal=Stafe_Relay_pin
  MeaModule1 : ec55xxlib/RapidECU_U2/11Calibration/MeaModule  signal=R2D_Voltage
  MeaModule2 : ec55xxlib/RapidECU_U2/11Calibration/MeaModule  signal=Buzzer_pin
  MeaModule3 : ec55xxlib/RapidECU_U2/11Calibration/MeaModule  signal=V48_relay
  MeaModule4 : ec55xxlib/RapidECU_U2/11Calibration/MeaModule  signal=IMD
  MeaModule5 : ec55xxlib/RapidECU_U2/11Calibration/MeaModule  signal=EBS
  MeaModule6 : ec55xxlib/RapidECU_U2/11Calibration/MeaModule  signal=BMS_LIGHT
  MeaModule7 : ec55xxlib/RapidECU_U2/11Calibration/MeaModule  signal=light_blue
  R2D_Pin : ec55xxlib/RapidECU_U2/04PowerDriverSwitch/PowerDriverSwitch  channel=118: O_PWM12_HS2A9  sampletime=-1
  "Safety_Relay " : ec55xxlib/RapidECU_U2/04PowerDriverSwitch/PowerDriverSwitch  channel=58: O_PWM1_LS1A8  sampletime=-1
  VCU_Valve : ec55xxlib/RapidECU_U2/04PowerDriverSwitch/PowerDriverSwitch  channel=61: O_PWM4_LS1A8  sampletime=-1
  VCU_Valve1 : ec55xxlib/RapidECU_U2/04PowerDriverSwitch/PowerDriverSwitch  channel=82: O_PWM5_LS1A8  sampletime=-1
  VCU_Valve2 : ec55xxlib/RapidECU_U2/04PowerDriverSwitch/PowerDriverSwitch  channel=90: O_PWM6_LS1A8  sampletime=-1
  VCU_Valve3 : ec55xxlib/RapidECU_U2/04PowerDriverSwitch/PowerDriverSwitch  channel=92: O_PWM7_LS1A8  sampletime=-1
  Yellow_Pin : ec55xxlib/RapidECU_U2/04PowerDriverSwitch/PowerDriverSwitch  channel=115: O_PWM10_HS2A9  sampletime=-1
  wires:
  Data Type Conversion1/1 -> Yellow_Pin/1
  VCU_valve/1 -> Data Type Conversion5/1
  Blue_Light_Pin/1 -> Data Type Conversion/1
  Buzzer_pin/1 -> Data Type Conversion2/1
  Data Type Conversion2/1 -> MeaModule2/1
  Data Type Conversion3/1 -> MeaModule/1
  Data Type Conversion4/1 -> MeaModule3/1
  Yellow_Light_Pin/1 -> Data Type Conversion1/1
  R2D_pin/1 -> Data Type Conversion6/1
  Data Type Conversion/1 -> MeaModule7/1
  Data Type Conversion9/1 -> MeaModule5/1
  MeaModule2/1 -> Buzzer_Pin/1
  EBS_Light/1 -> Data Type Conversion9/1
  BMS_Light/1 -> Data Type Conversion10/1
  Safety_Relay_Pin/1 -> Data Type Conversion3/1
  Data Type Conversion5/1 -> VCU_Valve/1
  MeaModule/1 -> "Safety_Relay "/1
  Data Type Conversion8/1 -> MeaModule4/1
  MeaModule4/1 -> VCU_Valve1/1
  MeaModule3/1 -> 48V_Relay/1
  MeaModule5/1 -> VCU_Valve2/1
  MeaModule6/1 -> VCU_Valve3/1
  IMD_Light/1 -> Data Type Conversion8/1
  Data Type Conversion6/1 -> MeaModule1/1
  Data Type Conversion10/1 -> MeaModule6/1
  MeaModule1/1 -> R2D_Pin/1
  Relay_48V_Pin/1 -> Data Type Conversion4/1
  MeaModule7/1 -> Blue_Pin/1
